simulink model "tank1"  (R2020b)
settings: Solver=VariableStepAuto  StartTime=0.0  StopTime=40000  RelTol=1e-3
values from neighbouring files (symbols this model uses):
  a_out = 0    [TankFillingScript.m]
  c = 16    [TankFillingScript.m]
  k_out = 0.1587/60    (= 0.002645)    [TankFillingScript.m]
settings Model: Creator=mreiff  LastModifiedBy=mreiff

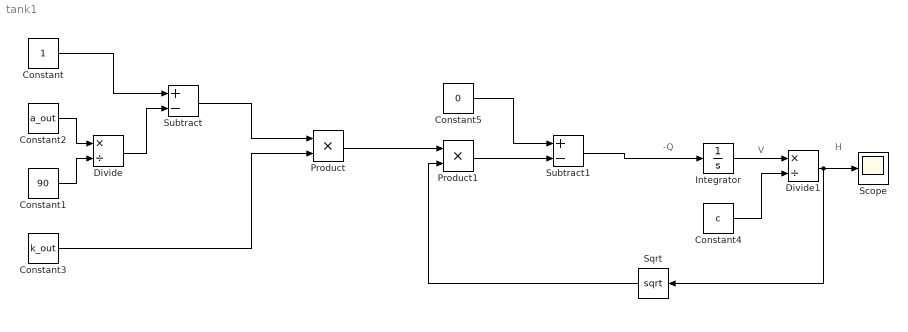
== system tank1 ==
  note: H
  note: V
  note: -Q
  Constant : Constant
  Constant1 : Constant  Value=90
  Constant2 : Constant  Value=a_out
  Constant3 : Constant  Value=k_out
  Constant4 : Constant  Value=c
  Constant5 : Constant  Value=0
  Divide : Product  Inputs=*/
  Divide1 : Product  Inputs=*/
  Integrator : Integrator  InitialCondition=64
  Product : Product
  Product1 : Product
  Scope : Scope
  Sqrt : Sqrt  SaturateOnIntegerOverflow=on
  Subtract : Sum  Inputs=+-
  Subtract1 : Sum  Inputs=+-
  wires:
  Constant2/1 -> Divide/1
  Constant1/1 -> Divide/2
  Divide/1 -> Subtract/2
  Constant/1 -> Subtract/1
  Constant3/1 -> Product/2
  Subtract/1 -> Product/1
  Product/1 -> Product1/1
  Integrator/1 -> Divide1/1
  Constant4/1 -> Divide1/2
  Divide1/1 -> Sqrt/1, Scope/1
  Sqrt/1 -> Product1/2
  Product1/1 -> Subtract1/2
  Subtract1/1 -> Integrator/1
  Constant5/1 -> Subtract1/1
